simulink library "aerolibactuator"  (Simulink 5.0)
settings Model: Creator=sgage  LastModifiedBy=sgage  ExtModeAutoUpdateStatusClock=off

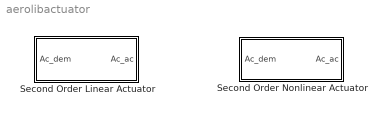
== system aerolibactuator ==
  Second Order Linear Actuator : Subsystem  mask(Second Order Linear Actuator){wn_fin=150, z_fin=0.7, fin_act_0=0}
      mask prompts: wn_fin "Natural frequency:"; z_fin "Damping ratio:"; fin_act_0 "Initial position:"
      mask help: Implement a second-order actuator model
      mask Help: web(asbhelp);
      mask Display:
      | port_label('input',1,'A_{demand}','texmode','on');
      | port_label('output',1,'A_{actual}','texmode','on');
  Second Order Nonlinear Actuator : Subsystem  mask(Second Order Nonlinear Actuator){wn_fin=150, z_fin=0.7, fin_max=20*pi/180, fin_min=-20*pi/180, fin_maxrate=500*pi/180, fin_act_0=0}
      mask prompts: wn_fin "Natural frequency:"; z_fin "Damping ratio:"; fin_max "Maximum deflection:"; fin_min "Minimum deflection:"; fin_maxrate "Maximum rate:"; fin_act_0 "Initial position:"
      mask help: Implement a second-order actuator model with saturation and rate limits.
      mask Help: web(asbhelp);
      mask Display:
      | port_label('input',1,'A_{demand}','texmode','on');
      | port_label('output',1,'A_{actual}','texmode','on');

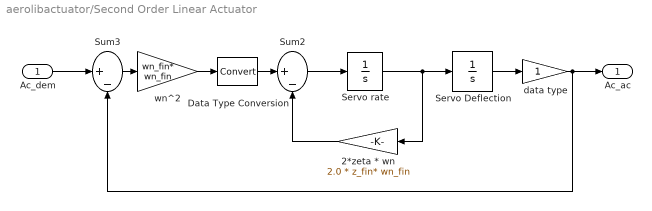
== system aerolibactuator/Second Order Linear Actuator ==
  Ac_dem : Inport
  2*zeta * wn : Gain  Orientation=left  Gain=2.0 * z_fin* wn_fin  SaturateOnIntegerOverflow=on
  Data Type Conversion : DataTypeConversion  SaturateOnIntegerOverflow=on
  Servo Deflection : Integrator  InitialCondition=fin_act_0  UpperSaturationLimit=Inf  LowerSaturationLimit=-Inf
  Servo rate : Integrator
  Sum2 : Sum  Inputs=|+-  SaturateOnIntegerOverflow=on  InputSameDT=on
  Sum3 : Sum  Inputs=|+-  SaturateOnIntegerOverflow=on  InputSameDT=on
  data type : Gain  ShowAdditionalParam=on  SaturateOnIntegerOverflow=on
  wn^2 : Gain  Gain=wn_fin* wn_fin  SaturateOnIntegerOverflow=on
  Ac_ac : Outport  InitialOutput=0
  wires:
  Data Type Conversion/1 -> Sum2/1
  data type/1 -> Sum3/2, Ac_ac/1
  Sum3/1 -> wn^2/1
  Ac_dem/1 -> Sum3/1
  2*zeta * wn/1 -> Sum2/2
  Servo rate/1 -> Servo Deflection/1, 2*zeta * wn/1
  Sum2/1 -> Servo rate/1
  wn^2/1 -> Data Type Conversion/1
  Servo Deflection/1 -> data type/1

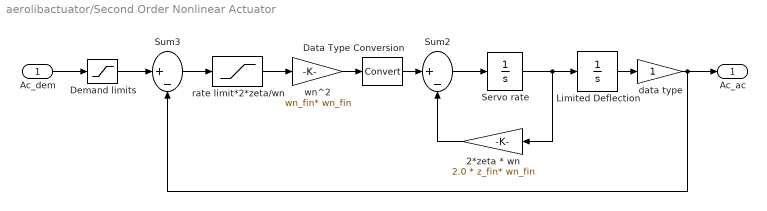
== system aerolibactuator/Second Order Nonlinear Actuator ==
  Ac_dem : Inport
  2*zeta * wn : Gain  Orientation=left  Gain=2.0 * z_fin* wn_fin  SaturateOnIntegerOverflow=on
  Data Type Conversion : DataTypeConversion  SaturateOnIntegerOverflow=on
  Demand limits : Saturate  UpperLimit=fin_max  LowerLimit=fin_min
  Limited Deflection : Integrator  InitialCondition=fin_act_0  LimitOutput=on  UpperSaturationLimit=fin_max  LowerSaturationLimit=fin_min
  Servo rate : Integrator
  Sum2 : Sum  Inputs=|+-  SaturateOnIntegerOverflow=on  InputSameDT=on
  Sum3 : Sum  Inputs=|+-  SaturateOnIntegerOverflow=on  InputSameDT=on
  data type : Gain  ShowAdditionalParam=on  SaturateOnIntegerOverflow=on
  rate limit*2*zeta/wn : Saturate  UpperLimit=fin_maxrate*2*z_fin/wn_fin  LowerLimit=-fin_maxrate*2*z_fin/wn_fin
  wn^2 : Gain  Gain=wn_fin* wn_fin  SaturateOnIntegerOverflow=on
  Ac_ac : Outport  InitialOutput=0
  wires:
  data type/1 -> Ac_ac/1, Sum3/2
  Data Type Conversion/1 -> Sum2/1
  Limited Deflection/1 -> data type/1
  wn^2/1 -> Data Type Conversion/1
  Sum2/1 -> Servo rate/1
  Servo rate/1 -> 2*zeta * wn/1, Limited Deflection/1
  2*zeta * wn/1 -> Sum2/2
  Sum3/1 -> rate limit*2*zeta/wn/1
  rate limit*2*zeta/wn/1 -> wn^2/1
  Demand limits/1 -> Sum3/1
  Ac_dem/1 -> Demand limits/1
